simulink model "sim_Prob4"  (R2023a)
settings: Solver=VariableStepAuto  StartTime=0.0  StopTime=N  RelTol=1e-3
undefined symbols (not defined in the file): denGdz, numGdz
settings Model: Creator=user  LastModifiedBy=user

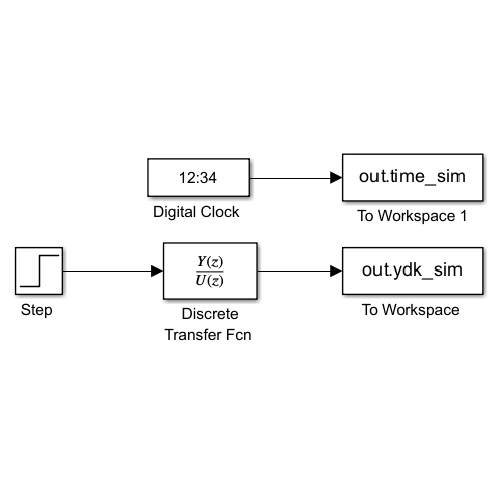
[thumbnail: Simulink's stored preview of the top-level diagram]
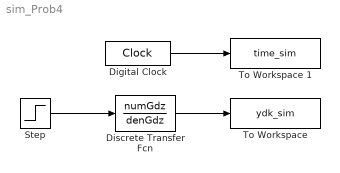
== system sim_Prob4 ==
  "Digital Clock " : DigitalClock  SampleTime=-1
  "Discrete Transfer Fcn " : DiscreteTransferFcn  Numerator=numGdz  Denominator=denGdz
  "Step " : Step  Time=0
  "To Workspace " : ToWorkspace  VariableName=ydk_sim  SampleTime=-1
  To Workspace 1 : ToWorkspace  VariableName=time_sim  SampleTime=-1
  wires:
  "Step "/1 -> "Discrete Transfer Fcn "/1
  "Discrete Transfer Fcn "/1 -> "To Workspace "/1
  "Digital Clock "/1 -> To Workspace 1/1
